simulink library "Pump_Simple"  (Simulink 8.2)
settings: Solver=ode45  StartTime=0.0  StopTime=10.0  RelTol=1e-3
libraries: carnot x1
settings Model: Creator=lena.frank  LastModifiedBy=drhf

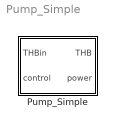
== system Pump_Simple ==
  Pump_Simple : Subsystem  mask(simple Pump){mdotmax=1200/3600, dia=0.0157, power=30, fluid_id=Water, mix=0, p0=3e5}
      mask prompts: mdotmax "massflow rate [kg/s]"; dia "diameter at in- and outlet [m]"; power "electric power consumption [W]"; fluid_id "fluid"; mix "percentage of fluid mix [0..1]"; p0 "system pressure [Pa]"
      mask help:
      | Set constant massflow rate according to the control signal.
      | The pump is a very basic model, sometimes creating algebraic loops. If you have problems with algebraic loops, use "Pump_const" instead.
      mask Help: web(fullfile(path_carnot('help'),'Pump_Const.html'),'-helpbrowser')
      mask TypeOptions fluid_id: Water | Air | Cotton Oil | Silicone Oil | Water-Glycol Mix | Tyfocor LS | Water (Constant 20°C) | Air (dry+ constant 20°C)
      mask Display:
      | plot(0,0,100,100,[40,70,40,30,30,40,60,70,70,60,40],[70,50,30,40,60,70,70,60,40,30,30])
      | port_label('input',1,'THB')
      | port_label('input',2,'ctr')
      | port_label('output',1,'THB')
      | port_label('output',2,'Pel')

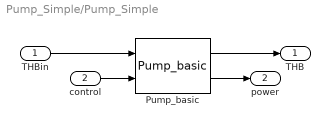
== system Pump_Simple/Pump_Simple ==
  THBin : Inport
  control : Inport  Port=2
  Pump_basic : carnot/Basic/Hydraulics/Pump_basic  mdotmax=mdotmax  fluid_id=fluid_id  mix=mix  dia=dia  power=power  p0=p0  hgt=0  ID=1
  THB : Outport
  power : Outport  Port=2
  wires:
  Pump_basic/2 -> power/1
  Pump_basic/1 -> THB/1
  control/1 -> Pump_basic/2
  THBin/1 -> Pump_basic/1
